simulink model "BicyclePathTracking1"  (R2026a)
settings: Solver=ode45  StopTime=30
StopFcn:
  | plot_bicycle_results;
libraries: slpidlib x1
settings Model: Creator=chitt  LastModifiedBy=chitt

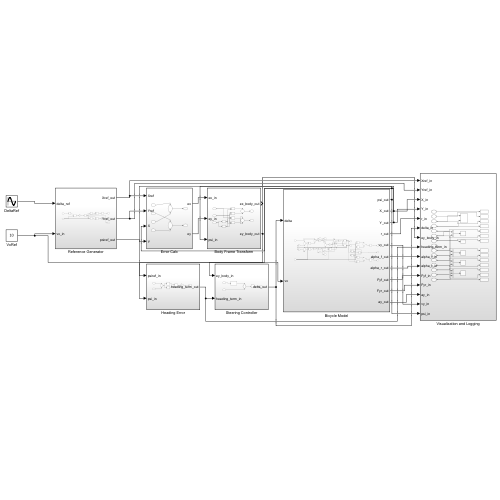
[thumbnail: Simulink's stored preview of the top-level diagram]
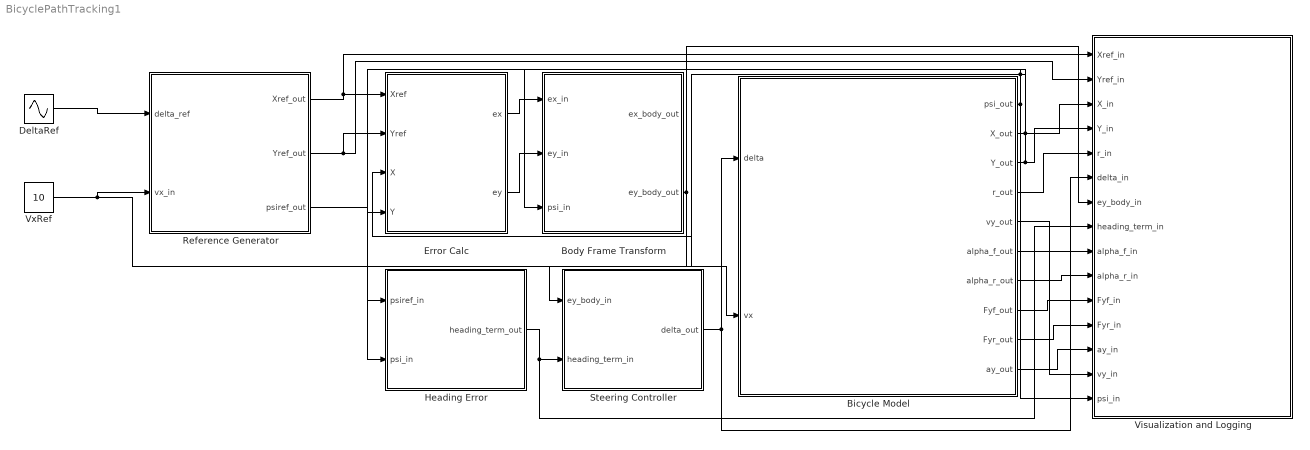
== system BicyclePathTracking1 ==
  Bicycle Model : Subsystem
  Body Frame Transform : Subsystem
  DeltaRef : Sin  Amplitude=0.08  Frequency=0.2  SampleTime=0
  Error Calc : Subsystem
  Heading Error : Subsystem
  Reference Generator : Subsystem
  Steering Controller : Subsystem
  Visualization and Logging : Subsystem
  VxRef : Constant  Value=10
  wires:
  DeltaRef/1 -> Reference Generator/1(delta_ref)
  VxRef/1 -> Reference Generator/2(vx_in), Bicycle Model/2(vx)
  Reference Generator/1(Xref_out) -> Error Calc/1(Xref), Visualization and Logging/1(Xref_in)
  Reference Generator/2(Yref_out) -> Error Calc/2(Yref), Visualization and Logging/2(Yref_in)
  Bicycle Model/2(X_out) -> Error Calc/3(X), Visualization and Logging/3(X_in)
  Bicycle Model/3(Y_out) -> Error Calc/4(Y), Visualization and Logging/4(Y_in)
  Error Calc/1(ex) -> Body Frame Transform/1(ex_in)
  Error Calc/2(ey) -> Body Frame Transform/2(ey_in)
  Bicycle Model/1(psi_out) -> Body Frame Transform/3(psi_in), Heading Error/2(psi_in), Visualization and Logging/15(psi_in)
  Reference Generator/3(psiref_out) -> Heading Error/1(psiref_in)
  Body Frame Transform/2(ey_body_out) -> Steering Controller/1(ey_body_in), Visualization and Logging/7(ey_body_in)
  Heading Error/1(heading_term_out) -> Steering Controller/2(heading_term_in), Visualization and Logging/8(heading_term_in)
  Steering Controller/1(delta_out) -> Bicycle Model/1(delta), Visualization and Logging/6(delta_in)
  Bicycle Model/4(r_out) -> Visualization and Logging/5(r_in)
  Bicycle Model/6(alpha_f_out) -> Visualization and Logging/9(alpha_f_in)
  Bicycle Model/7(alpha_r_out) -> Visualization and Logging/10(alpha_r_in)
  Bicycle Model/8(Fyf_out) -> Visualization and Logging/11(Fyf_in)
  Bicycle Model/9(Fyr_out) -> Visualization and Logging/12(Fyr_in)
  Bicycle Model/10(ay_out) -> Visualization and Logging/13(ay_in)
  Bicycle Model/5(vy_out) -> Visualization and Logging/14(vy_in)

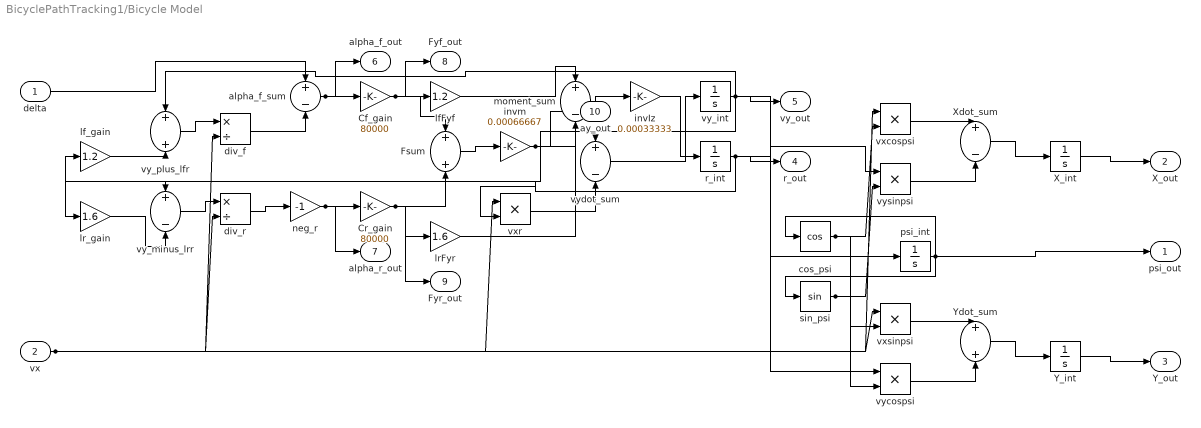
== system BicyclePathTracking1/Bicycle Model ==
  delta : Inport
  vx : Inport  Port=2
  Cf_gain : Gain  Gain=80000
  Cr_gain : Gain  Gain=80000
  Fsum : Sum
  X_int : Integrator
  Xdot_sum : Sum  Inputs=+-
  Y_int : Integrator
  Ydot_sum : Sum
  alpha_f_sum : Sum  Inputs=+-
  cos_psi : Trigonometry  Operator=cos
  div_f : Product  Inputs=*/
  div_r : Product  Inputs=*/
  invIz : Gain  Gain=0.00033333
  invm : Gain  Gain=0.00066667
  lfFyf : Gain  Gain=1.2
  lf_gain : Gain  Gain=1.2
  lrFyr : Gain  Gain=1.6
  lr_gain : Gain  Gain=1.6
  moment_sum : Sum  Inputs=+-
  neg_r : Gain  Gain=-1
  psi_int : Integrator
  r_int : Integrator
  sin_psi : Trigonometry
  vxcospsi : Product
  vxr : Product
  vxsinpsi : Product
  vy_int : Integrator
  vy_minus_lrr : Sum  Inputs=+-
  vy_plus_lfr : Sum
  vycospsi : Product
  vydot_sum : Sum  Inputs=+-
  vysinpsi : Product
  psi_out : Outport
  X_out : Outport  Port=2
  Y_out : Outport  Port=3
  r_out : Outport  Port=4
  vy_out : Outport  Port=5
  alpha_f_out : Outport  Port=6
  alpha_r_out : Outport  Port=7
  Fyf_out : Outport  Port=8
  Fyr_out : Outport  Port=9
  ay_out : Outport  Port=10
  wires:
  r_int/1 -> lf_gain/1, lr_gain/1, vxr/2, psi_int/1, r_out/1
  vy_int/1 -> vy_plus_lfr/1, vy_minus_lrr/1, vysinpsi/1, vycospsi/1, vy_out/1
  lf_gain/1 -> vy_plus_lfr/2
  vy_plus_lfr/1 -> div_f/1
  vx/1 -> div_f/2, div_r/2, vxr/1, vxcospsi/1, vxsinpsi/1
  delta/1 -> alpha_f_sum/1
  div_f/1 -> alpha_f_sum/2
  lr_gain/1 -> vy_minus_lrr/2
  vy_minus_lrr/1 -> div_r/1
  div_r/1 -> neg_r/1
  alpha_f_sum/1 -> Cf_gain/1, alpha_f_out/1
  neg_r/1 -> Cr_gain/1, alpha_r_out/1
  Cf_gain/1 -> Fsum/1, lfFyf/1, Fyf_out/1
  Cr_gain/1 -> Fsum/2, lrFyr/1, Fyr_out/1
  Fsum/1 -> invm/1
  invm/1 -> vydot_sum/1, ay_out/1
  vxr/1 -> vydot_sum/2
  vydot_sum/1 -> vy_int/1
  lfFyf/1 -> moment_sum/1
  lrFyr/1 -> moment_sum/2
  moment_sum/1 -> invIz/1
  invIz/1 -> r_int/1
  psi_int/1 -> cos_psi/1, sin_psi/1, psi_out/1
  cos_psi/1 -> vxcospsi/2, vycospsi/2
  sin_psi/1 -> vysinpsi/2, vxsinpsi/2
  vxcospsi/1 -> Xdot_sum/1
  vysinpsi/1 -> Xdot_sum/2
  Xdot_sum/1 -> X_int/1
  vxsinpsi/1 -> Ydot_sum/1
  vycospsi/1 -> Ydot_sum/2
  Ydot_sum/1 -> Y_int/1
  X_int/1 -> X_out/1
  Y_int/1 -> Y_out/1

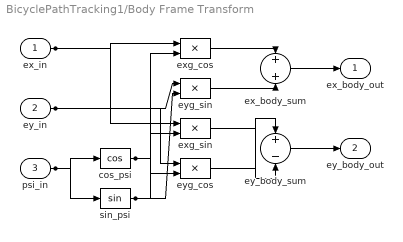
== system BicyclePathTracking1/Body Frame Transform ==
  ex_in : Inport
  ey_in : Inport  Port=2
  psi_in : Inport  Port=3
  cos_psi : Trigonometry  Operator=cos
  ex_body_sum : Sum
  exg_cos : Product
  exg_sin : Product
  ey_body_sum : Sum  Inputs=+-
  eyg_cos : Product
  eyg_sin : Product
  sin_psi : Trigonometry
  ex_body_out : Outport
  ey_body_out : Outport  Port=2
  wires:
  ex_in/1 -> exg_cos/1, exg_sin/1
  cos_psi/1 -> exg_cos/2, eyg_cos/2
  ey_in/1 -> eyg_sin/1, eyg_cos/1
  sin_psi/1 -> eyg_sin/2, exg_sin/2
  exg_cos/1 -> ex_body_sum/1
  eyg_sin/1 -> ex_body_sum/2
  eyg_cos/1 -> ey_body_sum/1
  exg_sin/1 -> ey_body_sum/2
  psi_in/1 -> cos_psi/1, sin_psi/1
  ex_body_sum/1 -> ex_body_out/1
  ey_body_sum/1 -> ey_body_out/1

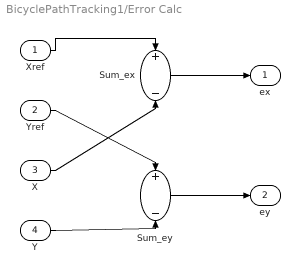
== system BicyclePathTracking1/Error Calc ==
  Xref : Inport
  Yref : Inport  Port=2
  X : Inport  Port=3
  Y : Inport  Port=4
  Sum_ex : Sum  Inputs=+-
  Sum_ey : Sum  Inputs=+-
  ex : Outport
  ey : Outport  Port=2
  wires:
  Xref/1 -> Sum_ex/1
  X/1 -> Sum_ex/2
  Sum_ex/1 -> ex/1
  Yref/1 -> Sum_ey/1
  Y/1 -> Sum_ey/2
  Sum_ey/1 -> ey/1

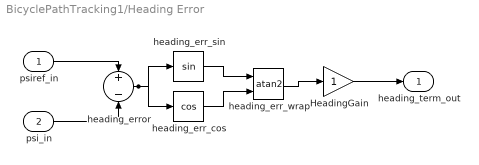
== system BicyclePathTracking1/Heading Error ==
  psiref_in : Inport
  psi_in : Inport  Port=2
  HeadingGain : Gain
  heading_err_cos : Trigonometry  Operator=cos
  heading_err_sin : Trigonometry
  heading_err_wrap : Trigonometry  Operator=atan2
  heading_error : Sum  Inputs=+-
  heading_term_out : Outport
  wires:
  psiref_in/1 -> heading_error/1
  psi_in/1 -> heading_error/2
  heading_error/1 -> heading_err_sin/1, heading_err_cos/1
  heading_err_sin/1 -> heading_err_wrap/1
  heading_err_cos/1 -> heading_err_wrap/2
  heading_err_wrap/1 -> HeadingGain/1
  HeadingGain/1 -> heading_term_out/1

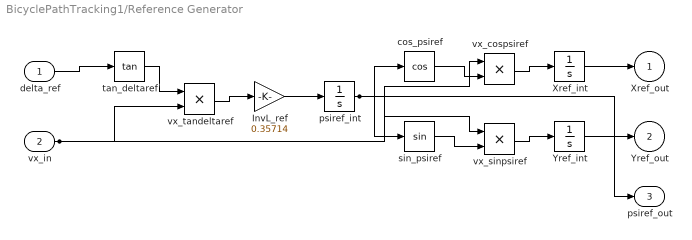
== system BicyclePathTracking1/Reference Generator ==
  delta_ref : Inport
  vx_in : Inport  Port=2
  InvL_ref : Gain  Gain=0.35714
  Xref_int : Integrator
  Yref_int : Integrator
  cos_psiref : Trigonometry  Operator=cos
  psiref_int : Integrator
  sin_psiref : Trigonometry
  tan_deltaref : Trigonometry  Operator=tan
  vx_cospsiref : Product
  vx_sinpsiref : Product
  vx_tandeltaref : Product
  Xref_out : Outport
  Yref_out : Outport  Port=2
  psiref_out : Outport  Port=3
  wires:
  delta_ref/1 -> tan_deltaref/1
  tan_deltaref/1 -> vx_tandeltaref/1
  vx_in/1 -> vx_tandeltaref/2, vx_cospsiref/1, vx_sinpsiref/1
  vx_tandeltaref/1 -> InvL_ref/1
  InvL_ref/1 -> psiref_int/1
  psiref_int/1 -> cos_psiref/1, sin_psiref/1, psiref_out/1
  cos_psiref/1 -> vx_cospsiref/2
  vx_cospsiref/1 -> Xref_int/1
  sin_psiref/1 -> vx_sinpsiref/2
  vx_sinpsiref/1 -> Yref_int/1
  Xref_int/1 -> Xref_out/1
  Yref_int/1 -> Yref_out/1

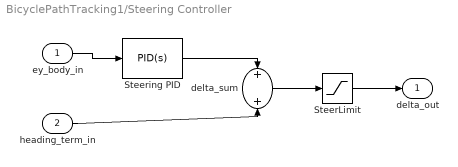
== system BicyclePathTracking1/Steering Controller ==
  ey_body_in : Inport
  heading_term_in : Inport  Port=2
  SteerLimit : Saturate
  Steering PID : slpidlib/PID Controller  Controller=PID  Form=Parallel  TimeDomain=Continuous-time  UseExternalTs=off  SampleTime=-1  IntegratorMethod=Forward Euler  FilterMethod=Forward Euler  ControllerParametersSource=internal  P=0.8  I=0.05  UseKiTs=off  D=0.05  UseExternalDerivativeSource=off  N=100  UseFilter=on  TunerSelectOption=Transfer Function Based (PID Tuner App)  InitialConditionSource=internal  InitialConditionForIntegrator=0  InitialConditionForFilter=0  DifferentiatorICPrevScaledInput=0  ExternalReset=none  TrackingMode=off  Kt=1  LimitOutput=off  SatLimitsSource=internal  UpperSaturationLimit=inf  LowerSaturationLimit=-inf  LinearizeAsGain=on  AntiWindupMode=none  Kb=1  LimitIntegrator=off  UpperIntegratorSaturationLimit=inf  LowerIntegratorSaturationLimit=-inf  POutMin=[]  POutMax=[]  IOutMin=[]  IOutMax=[]  DOutMin=[]  DOutMax=[]  NOutMin=[]  NOutMax=[]  SumOutMin=[]  SumOutMax=[]  SaturationOutMin=[]  SaturationOutMax=[]  PParamMin=[]  PParamMax=[]  IParamMin=[]  IParamMax=[]  DParamMin=[]  DParamMax=[]  NParamMin=[]  NParamMax=[]  KbParamMin=[]  KbParamMax=[]  KtParamMin=[]  KtParamMax=[]  KbOutMin=[]  KbOutMax=[]  KtOutMin=[]  KtOutMax=[]  IntegratorOutMin=[]  IntegratorOutMax=[]  FilterOutMin=[]  FilterOutMax=[]  SumI1OutMin=[]  SumI1OutMax=[]  SumI2OutMin=[]  SumI2OutMax=[]  SumI3OutMin=[]  SumI3OutMax=[]  SumI4OutMin=[]  SumI4OutMax=[]  SumDOutMin=[]  SumDOutMax=[]  DifferentiatorOutMin=[]  DifferentiatorOutMax=[]  FilterDiffOutCoefMin=[]  FilterDiffOutCoefMax=[]  ReciprocalOutMin=[]  ReciprocalOutMax=[]  SumDenOutMin=[]  SumDenOutMax=[]  SumNumOutMin=[]  SumNumOutMax=[]  DivideOutMin=[]  DivideOutMax=[]  UdiffTsProdOutMin=[]  UdiffTsProdOutMax=[]  NTsProdOutMin=[]  NTsProdOutMax=[]  UintegralTsProdOutMin=[]  UintegralTsProdOutMax=[]  UngainTsProdOutMin=[]  UngainTsProdOutMax=[]  ClampingZeroOutDataTypeStr=Inherit: Inherit via back propagation  ClampingZeroOutMin=[]  ClampingZeroOutMax=[]  FilterDenConstantOutDataTypeStr=Inherit: Inherit via back propagation  FilterDenConstantOutMin=[]  FilterDenConstantOutMax=[]  PCopyOutDataTypeStr=Inherit: Inherit via back propagation  PCopyOutMin=[]  PCopyOutMax=[]  NCopyOutDataTypeStr=Inherit: Inherit via back propagation  NCopyOutMin=[]  NCopyOutMax=[]  IntegratorContinuousStateAttributes=''  IntegratorStateMustResolveToSignalObject=off  IntegratorRTWStateStorageClass=Auto  FilterContinuousStateAttributes=''  FilterStateMustResolveToSignalObject=off  FilterRTWStateStorageClass=Auto  ParallelPVariant=InternalParameters  IdealPVariant=Disabled  IVariant=InternalParameters  DVariant=InternalParameters  IntegratorVariant=Continuous  SatVariant=Disabled  AWVariant=Passthrough  PCopyVariant=Disabled  TRVariant=Disabled  FdbkBlocksVariant=Forward  IdealPFdbkVariant=Disabled  SatFdbkVariant=Disabled  DerivativeFilterVariant=ContFilter  NVariant=InternalParameters  NCopyVariant=Disabled  FilterICVariant=InternalICsFilter  IntegratorICVariant=InternalICs  ExternalResetVariant=Disabled  TRSumVariant=Passthrough  SumFdbkVariant=Disabled  SumVariant=Sum_PID  TsampFilterVariant=InternalTs  TsampNgainVariant=Passthrough  TsampIntegralVariant=Disabled_SignalSpec  ExternalSaturationOutDataTypeStr=Inherit: Same as second input  DerivativeSourceVariant=ErrorSignal  PreIntVariant=InternalPreInt
  delta_sum : Sum
  delta_out : Outport
  wires:
  ey_body_in/1 -> Steering PID/1
  Steering PID/1 -> delta_sum/1
  heading_term_in/1 -> delta_sum/2
  delta_sum/1 -> SteerLimit/1
  SteerLimit/1 -> delta_out/1

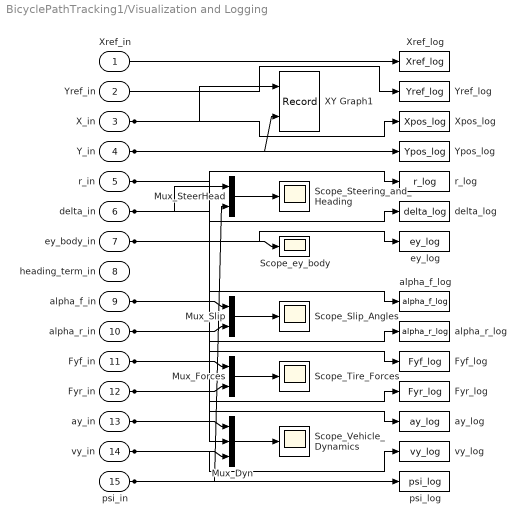
== system BicyclePathTracking1/Visualization and Logging ==
  Xref_in : Inport
  Yref_in : Inport  Port=2
  X_in : Inport  Port=3
  Y_in : Inport  Port=4
  r_in : Inport  Port=5
  delta_in : Inport  Port=6
  ey_body_in : Inport  Port=7
  heading_term_in : Inport  Port=8
  alpha_f_in : Inport  Port=9
  alpha_r_in : Inport  Port=10
  Fyf_in : Inport  Port=11
  Fyr_in : Inport  Port=12
  ay_in : Inport  Port=13
  vy_in : Inport  Port=14
  psi_in : Inport  Port=15
  Fyf_log : ToWorkspace  VariableName=Fyf_log  SaveFormat=Timeseries  SampleTime=-1
  Fyr_log : ToWorkspace  VariableName=Fyr_log  SaveFormat=Timeseries  SampleTime=-1
  Mux_Dyn : Mux  Inputs=3
  Mux_Forces : Mux  Inputs=2
  Mux_Slip : Mux  Inputs=2
  Mux_SteerHead : Mux  Inputs=2
  Scope_Slip_Angles : Scope
  Scope_Steering_and_Heading : Scope
  Scope_Tire_Forces : Scope
  Scope_Vehicle_Dynamics : Scope
  Scope_ey_body : Scope
  XY Graph1 : Record  NumPorts=2.0  FileSettingsInternal="{\"entries\":[{\"content\":{\"excelSettings\":{\"content\":{},\"type\":\"Streamout.ExcelSettings\"},\"parquetSettings\":{\"content\":{},\"type\":\"Streamout.ParquetSettings\"}},\"type\":\"Streamout.FileSettingStorage\",\"uuid\":\"\"}],\"packageUris\":[\"http:\\/\\/schema.mathworks.com\\/mf0\\/streamout_blocks\\/R2020a\"],\"version\":\"1.0\"}"  FrameSettings=[0, 0]  Layout=[1 1]  SignalsInternal="{\"entries\":[{\"content\":{\"signals\":[{\"content\":{\"blockPath\":[],\"dimensions\":[1],\"domain\":\"\",\"lineColor\":\"#a2142f\",\"plots\":[ 1 ],\"port\":1,\"sid\":[\"\"],\"signalID\":1,\"signalName\":\"X_in\"},\"type\":\"RecordBlkView.Signal\",\"uuid\":\"\"},{\"content\":{\"blockPath\":[],\"dimensions\":[1],\"domain\":\"\",\"lineColor\":\"#139fff\",\"plots\":[ 1 ],\"port\":2,\"sid\":[\"\"],\"signalID\":2,\"signalName\":\"Y_in\"},\"type\":\"RecordBlkView.Signal\",\"uuid\":\"\"}]},\"type\":\"RecordBlkView.InputSignals\",\"uuid\":\"\"}],\"packageUris\":[\"http:\\/\\/schema.mathworks.com\\/mf0\\/streamout_blocks\\/R2020a\"],\"version\":\"1.0\"}"  VisualizationBindings="{\"xyplotplugin\":{\"info\":[{\"series\":[{\"bindingParametersList\":[{\"parameter\":\"X-Axis\",\"signalID\":1,\"signalName\":\"X_in\"},{\"parameter\":\"Y-Axis\",\"signalID\":2,\"signalName\":\"Y_in\"}],\"seriesID\":0}],\"subplotID\":1}]}}"  CompatibilityTag=XY
  Xpos_log : ToWorkspace  VariableName=Xpos_log  SaveFormat=Timeseries  SampleTime=-1
  Xref_log : ToWorkspace  VariableName=Xref_log  SaveFormat=Timeseries  SampleTime=-1
  Ypos_log : ToWorkspace  VariableName=Ypos_log  SaveFormat=Timeseries  SampleTime=-1
  Yref_log : ToWorkspace  VariableName=Yref_log  SaveFormat=Timeseries  SampleTime=-1
  alpha_f_log : ToWorkspace  VariableName=alpha_f_log  SaveFormat=Timeseries  SampleTime=-1
  alpha_r_log : ToWorkspace  VariableName=alpha_r_log  SaveFormat=Timeseries  SampleTime=-1
  ay_log : ToWorkspace  VariableName=ay_log  SaveFormat=Timeseries  SampleTime=-1
  delta_log : ToWorkspace  VariableName=delta_log  SaveFormat=Timeseries  SampleTime=-1
  ey_log : ToWorkspace  VariableName=ey_log  SaveFormat=Timeseries  SampleTime=-1
  psi_log : ToWorkspace  VariableName=psi_log  SaveFormat=Timeseries  SampleTime=-1
  r_log : ToWorkspace  VariableName=r_log  SaveFormat=Timeseries  SampleTime=-1
  vy_log : ToWorkspace  VariableName=vy_log  SaveFormat=Timeseries  SampleTime=-1
  wires:
  delta_in/1 -> Mux_SteerHead/1, delta_log/1
  psi_in/1 -> Mux_SteerHead/2, psi_log/1
  Mux_SteerHead/1 -> Scope_Steering_and_Heading/1
  alpha_f_in/1 -> Mux_Slip/1, alpha_f_log/1
  alpha_r_in/1 -> Mux_Slip/2, alpha_r_log/1
  Mux_Slip/1 -> Scope_Slip_Angles/1
  Fyf_in/1 -> Mux_Forces/1, Fyf_log/1
  Fyr_in/1 -> Mux_Forces/2, Fyr_log/1
  Mux_Forces/1 -> Scope_Tire_Forces/1
  ay_in/1 -> Mux_Dyn/1, ay_log/1
  r_in/1 -> Mux_Dyn/2, r_log/1
  vy_in/1 -> Mux_Dyn/3, vy_log/1
  Mux_Dyn/1 -> Scope_Vehicle_Dynamics/1
  ey_body_in/1 -> Scope_ey_body/1, ey_log/1
  X_in/1 -> XY Graph1/1, Xpos_log/1
  Y_in/1 -> XY Graph1/2, Ypos_log/1
  Xref_in/1 -> Xref_log/1
  Yref_in/1 -> Yref_log/1
